simulink model "electromech_dynamics_debug"  (R2020b)
settings: Solver=ode3  StartTime=0.0  StopTime=10.0  RelTol=1e-3
undefined symbols (not defined in the file or in its folder): C12qq_coeff, Fv1, g2_coeff, M11q, M12q_coeff, M22q, ua2tau1
settings Model: Creator=gioel  LastModifiedBy=gioel

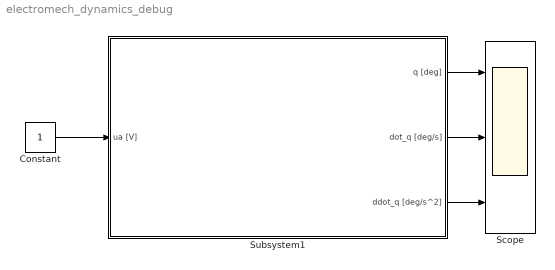
== system electromech_dynamics_debug ==
  Constant : Constant
  Scope : Scope  NumInputPorts=3
  Subsystem1 : Subsystem
  wires:
  Constant/1 -> Subsystem1/1(ua [V])
  Subsystem1/1(q [deg]) -> Scope/1
  Subsystem1/2(dot_q [deg/s]) -> Scope/2
  Subsystem1/3(ddot_q [deg/s^2]) -> Scope/3

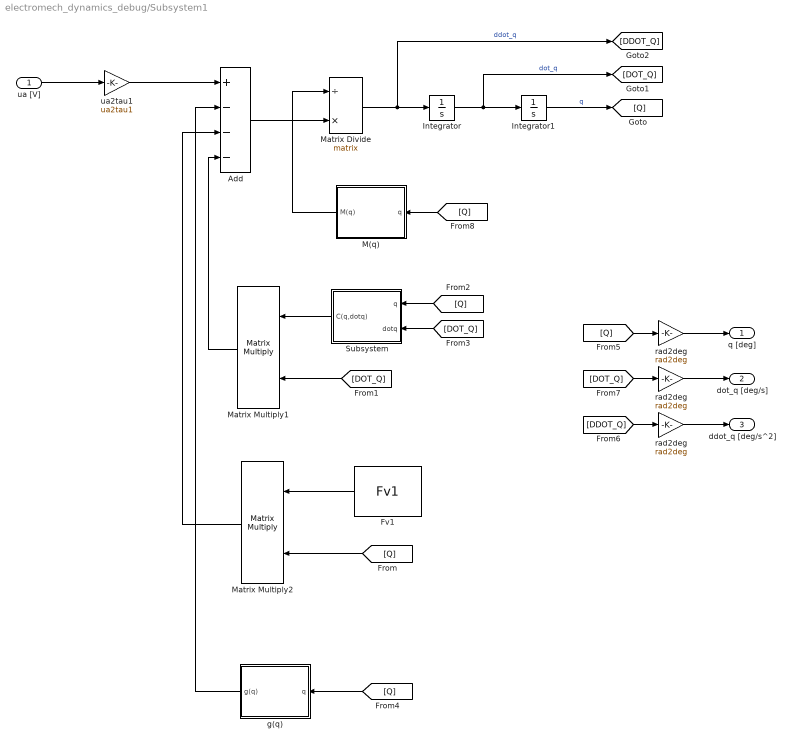
== system electromech_dynamics_debug/Subsystem1 ==
  ua [V] : Inport
  Add : Sum  Inputs=+---
  Fv1 : Constant  Value=Fv1
  Integrator : Integrator
  Integrator1 : Integrator
  M(q) : Subsystem
  Matrix Divide : Product  Inputs=/*  Multiplication=Matrix(*)
  Matrix Multiply1 : Product  Multiplication=Matrix(*)
  Matrix Multiply2 : Product  Multiplication=Matrix(*)
  Subsystem : Subsystem
  g(q) : Subsystem
  rad2deg : Gain  Gain=rad2deg
  "rad2deg " : Gain  Gain=rad2deg
  "rad2deg  " : Gain  Gain=rad2deg
  ua2tau1 : Gain  Gain=ua2tau1
  q [deg] : Outport
  dot_q [deg/s] : Outport  Port=2
  ddot_q [deg/s^2] : Outport  Port=3
  wires:
  ua2tau1/1 -> Add/1
  Integrator/1 -> [DOT_Q], Integrator1/1  "dot_q"
  g(q)/1(g(q)) -> Add/2
  M(q)/1(M(q)) -> Matrix Divide/1
  [DOT_Q] -> "rad2deg  "/1
  Matrix Multiply2/1 -> Add/3
  [DOT_Q] -> Subsystem/2(dotq)
  [Q] -> Matrix Multiply2/2
  Add/1 -> Matrix Divide/2
  Fv1/1 -> Matrix Multiply2/1
  [DOT_Q] -> Matrix Multiply1/2
  Matrix Multiply1/1 -> Add/4
  [DDOT_Q] -> "rad2deg "/1
  Matrix Divide/1 -> [DDOT_Q], Integrator/1  "ddot_q"
  [Q] -> Subsystem/1(q)
  Subsystem/1(C(q,dotq)) -> Matrix Multiply1/1
  [Q] -> rad2deg/1
  [Q] -> M(q)/1(q)
  Integrator1/1 -> [Q]  "q"
  "rad2deg  "/1 -> dot_q [deg/s]/1
  ua [V]/1 -> ua2tau1/1
  rad2deg/1 -> q [deg]/1
  "rad2deg "/1 -> ddot_q [deg/s^2]/1
  [Q] -> g(q)/1(q)

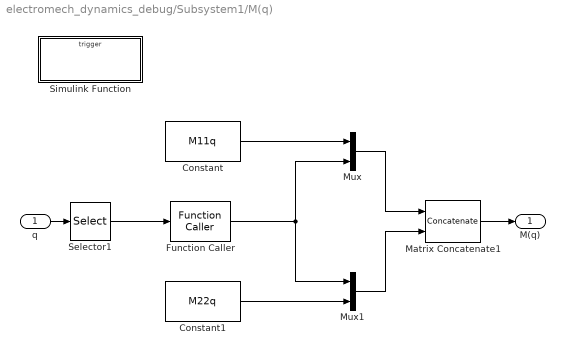
== system electromech_dynamics_debug/Subsystem1/M(q) ==
  q : Inport
  Constant : Constant  Value=M11q
  Constant1 : Constant  Value=M22q
  Function Caller : FunctionCaller  FunctionPrototype=y = M12q(u)  InputArgumentSpecifications=<Enter example>  OutputArgumentSpecifications=<Enter example>
  Matrix Concatenate1 : Concatenate  Mode=Multidimensional array  ConcatenateDimension=2
  Mux : Mux  Inputs=2
  Mux1 : Mux  Inputs=2
  Selector1 : Selector  InputPortWidth=2  IndexOptions=Index vector (dialog)  Indices=2  OutputSizes=1
  Simulink Function : Subsystem  TreatAsAtomicUnit=on
  M(q) : Outport
  wires:
  q/1 -> Selector1/1
  Mux1/1 -> Matrix Concatenate1/2
  Constant1/1 -> Mux1/2
  Mux/1 -> Matrix Concatenate1/1
  Function Caller/1 -> Mux/2, Mux1/1
  Matrix Concatenate1/1 -> M(q)/1
  Selector1/1 -> Function Caller/1
  Constant/1 -> Mux/1

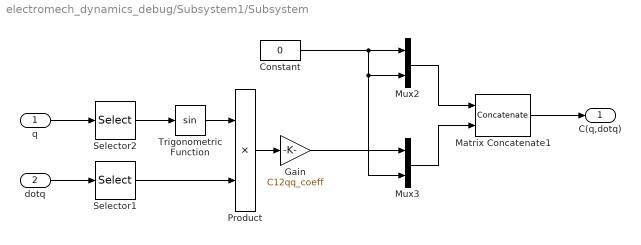
== system electromech_dynamics_debug/Subsystem1/Subsystem ==
  q : Inport
  dotq : Inport  Port=2
  Constant : Constant  Value=0
  Gain : Gain  Gain=C12qq_coeff
  Matrix Concatenate1 : Concatenate  Mode=Multidimensional array  ConcatenateDimension=2
  Mux2 : Mux  Inputs=2
  Mux3 : Mux  Inputs=2
  Product : Product
  Selector1 : Selector  InputPortWidth=2  IndexOptions=Index vector (dialog)  Indices=2  OutputSizes=1
  Selector2 : Selector  InputPortWidth=2  IndexOptions=Index vector (dialog)  Indices=2  OutputSizes=1
  Trigonometric Function : Trigonometry
  C(q,dotq) : Outport
  wires:
  Mux3/1 -> Matrix Concatenate1/2
  Mux2/1 -> Matrix Concatenate1/1
  Constant/1 -> Mux3/2, Mux2/2, Mux2/1
  Matrix Concatenate1/1 -> C(q,dotq)/1
  Gain/1 -> Mux3/1
  q/1 -> Selector2/1
  dotq/1 -> Selector1/1
  Selector1/1 -> Product/2
  Product/1 -> Gain/1
  Trigonometric Function/1 -> Product/1
  Selector2/1 -> Trigonometric Function/1

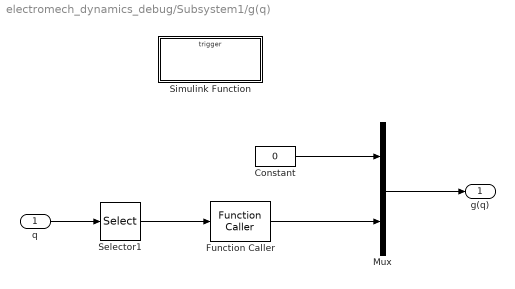
== system electromech_dynamics_debug/Subsystem1/g(q) ==
  q : Inport
  Constant : Constant  Value=0
  Function Caller : FunctionCaller  FunctionPrototype=y = g2(u)  InputArgumentSpecifications=<Enter example>  OutputArgumentSpecifications=<Enter example>
  Mux : Mux  Inputs=2
  Selector1 : Selector  InputPortWidth=2  IndexOptions=Index vector (dialog)  Indices=2  OutputSizes=1
  Simulink Function : Subsystem  TreatAsAtomicUnit=on
  g(q) : Outport
  wires:
  q/1 -> Selector1/1
  Selector1/1 -> Function Caller/1
  Constant/1 -> Mux/1
  Function Caller/1 -> Mux/2
  Mux/1 -> g(q)/1

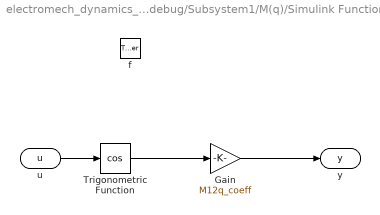
== system electromech_dynamics_debug/Subsystem1/M(q)/Simulink Function ==
  f : TriggerPort  TriggerType=function-call  IsSimulinkFunction=on  FunctionName=M12q  FunctionVisibility=scoped  VariantControl=(inherit)
  Gain : Gain  Gain=M12q_coeff
  Trigonometric Function : Trigonometry  Operator=cos
  u : ArgIn  DisableCoverage=on  ArgumentName=u
  y : ArgOut  DisableCoverage=on  ArgumentName=y
  wires:
  u/1 -> Trigonometric Function/1
  Trigonometric Function/1 -> Gain/1
  Gain/1 -> y/1

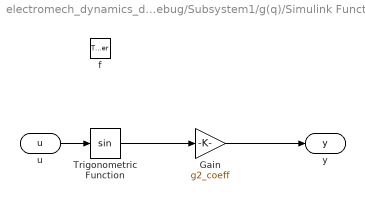
== system electromech_dynamics_debug/Subsystem1/g(q)/Simulink Function ==
  f : TriggerPort  TriggerType=function-call  IsSimulinkFunction=on  FunctionName=g2  FunctionVisibility=scoped  VariantControl=(inherit)
  Gain : Gain  Gain=g2_coeff
  Trigonometric Function : Trigonometry
  u : ArgIn  DisableCoverage=on  ArgumentName=u
  y : ArgOut  DisableCoverage=on  ArgumentName=y
  wires:
  u/1 -> Trigonometric Function/1
  Trigonometric Function/1 -> Gain/1
  Gain/1 -> y/1
